simulink model "task2_lab14"  (R2021a)
settings: Solver=VariableStepAuto  StartTime=0.0  StopTime=10.0  RelTol=1e-3
settings Model: Creator=reemb  LastModifiedBy=reemb

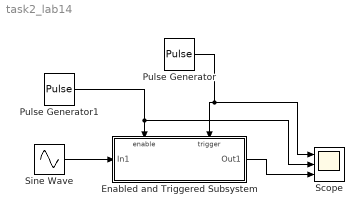
== system task2_lab14 ==
  Enabled and Triggered Subsystem : Subsystem  TreatAsAtomicUnit=on
  Pulse Generator : DiscretePulseGenerator  PulseType=Time based  Period=1  PulseWidth=50
  Pulse Generator1 : DiscretePulseGenerator  PulseType=Time based  Period=4  PulseWidth=50
  Scope : Scope  NumInputPorts=3
  Sine Wave : Sin  SampleTime=0
  wires:
  Pulse Generator1/1 -> Scope/2, Enabled and Triggered Subsystem/Enable
  Enabled and Triggered Subsystem/1(Out1) -> Scope/3
  Pulse Generator/1 -> Scope/1, Enabled and Triggered Subsystem/Trigger
  Sine Wave/1 -> Enabled and Triggered Subsystem/1(In1)

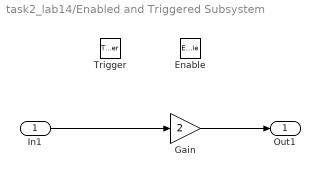
== system task2_lab14/Enabled and Triggered Subsystem ==
  In1 : Inport
  Enable : EnablePort
  Trigger : TriggerPort  VariantControl=(inherit)
  Gain : Gain  Gain=2
  Out1 : Outport
  wires:
  In1/1 -> Gain/1
  Gain/1 -> Out1/1
